simulink model "LQR_sim_with_equations_of_motion"  (R2022b)
settings: Solver=VariableStepAuto  StartTime=0.0  StopTime=10  RelTol=1e-3
undefined symbols (not defined in the file or in its folder): DiscIntNeverNeededParam, K
settings Model: Creator=Edvin  LastModifiedBy=Edvin

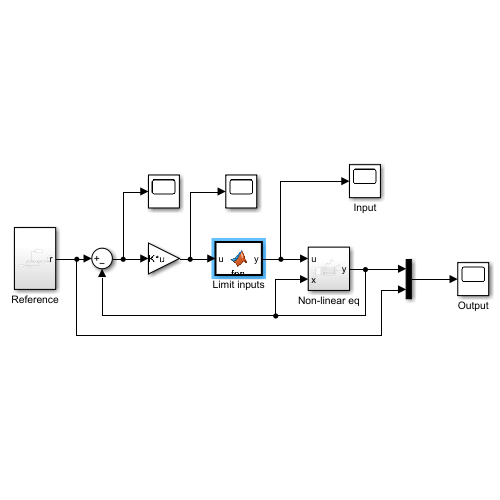
[thumbnail: Simulink's stored preview of the top-level diagram]
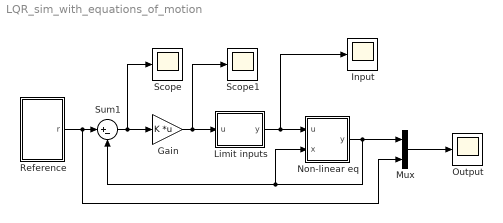
== system LQR_sim_with_equations_of_motion ==
  Gain : Gain  Gain=K  Multiplication=Matrix(K*u)
  Input : Scope
  Limit inputs : MATLAB Function  TreatAsAtomicUnit=on
  Mux : Mux  Inputs=2
  Non-linear eq : Subsystem
  Output : Scope
  Reference : Subsystem
  Scope : Scope
  Scope1 : Scope
  Sum1 : Sum  Inputs=|+-
  wires:
  Sum1/1 -> Scope/1, Gain/1
  Mux/1 -> Output/1
  Non-linear eq/1(y) -> Sum1/2, Non-linear eq/2(x), Mux/1
  Gain/1 -> Scope1/1, Limit inputs/1(u)
  Reference/1(r) -> Mux/2, Sum1/1
  Limit inputs/1(y) -> Input/1, Non-linear eq/1(u)

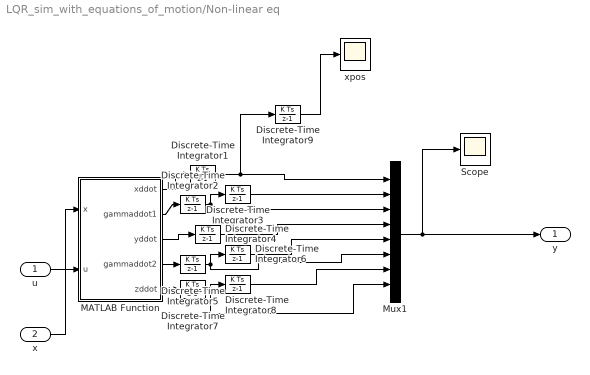
== system LQR_sim_with_equations_of_motion/Non-linear eq ==
  u : Inport
  x : Inport  Port=2
  Discrete-Time Integrator{1..9} (9 alike) : DiscreteIntegrator  SampleTime=-1  ICPrevOutput=DiscIntNeverNeededParam  ICPrevScaledInput=DiscIntNeverNeededParam
  MATLAB Function : MATLAB Function  TreatAsAtomicUnit=on
  Mux1 : Mux  Inputs=8
  Scope : Scope
  xpos : Scope
  y : Outport
  wires:
  MATLAB Function/1(xddot) -> Discrete-Time Integrator1/1
  u/1 -> MATLAB Function/2(u)
  Discrete-Time Integrator2/1 -> Mux1/3, Discrete-Time Integrator3/1
  MATLAB Function/2(gammaddot1) -> Discrete-Time Integrator2/1
  Discrete-Time Integrator6/1 -> Mux1/5
  MATLAB Function/3(yddot) -> Discrete-Time Integrator4/1
  Discrete-Time Integrator1/1 -> Discrete-Time Integrator9/1, Mux1/1
  MATLAB Function/5(zddot) -> Discrete-Time Integrator7/1
  Discrete-Time Integrator4/1 -> Mux1/4
  MATLAB Function/4(gammaddot2) -> Discrete-Time Integrator5/1
  Discrete-Time Integrator8/1 -> Mux1/7
  x/1 -> MATLAB Function/1(x)
  Discrete-Time Integrator5/1 -> Discrete-Time Integrator6/1, Mux1/6
  Discrete-Time Integrator3/1 -> Mux1/2
  Discrete-Time Integrator7/1 -> Discrete-Time Integrator8/1, Mux1/8
  Discrete-Time Integrator9/1 -> xpos/1
  Mux1/1 -> y/1, Scope/1

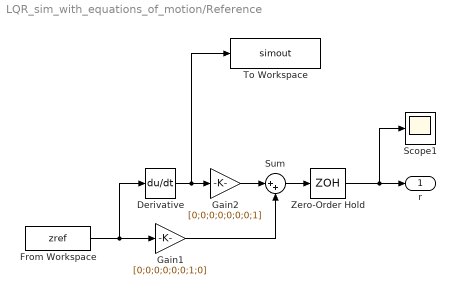
== system LQR_sim_with_equations_of_motion/Reference ==
  Derivative : Derivative
  From Workspace : FromWorkspace  VariableName=zref
  Gain1 : Gain  Gain=[0;0;0;0;0;0;1;0]
  Gain2 : Gain  Gain=[0;0;0;0;0;0;0;1]
  Scope1 : Scope
  Sum : Sum  Inputs=|++
  To Workspace : ToWorkspace  VariableName=simout  SampleTime=-1
      settings: Save2DSignal=2-D array (concatenate along first dimension)
  Zero-Order Hold : ZeroOrderHold  SampleTime=0.01
  r : Outport
  wires:
  Derivative/1 -> Gain2/1, To Workspace/1
  From Workspace/1 -> Derivative/1, Gain1/1
  Sum/1 -> Zero-Order Hold/1
  Gain1/1 -> Sum/2
  Gain2/1 -> Sum/1
  Zero-Order Hold/1 -> r/1, Scope1/1

== matlab function LQR_sim_with_equations_of_motion/Limit inputs ==
  data: u input; y output
function y = fcn(u)
g = 9.82; 
m = 2.5;
% Max thrust
Fmax = m*g;

% Calculate thrust
u(1) = m*g/2 + u(1);

% Limit thrust vector
if u(1) > Fmax
    u(1) = Fmax;
elseif u(1) <= 0 
    u(1) = 0;
end

% Limit gimble angles
if u(2) > 30
    u(2) = 30;
elseif u(2) < -30
    u(2) = -30;
end

if u(3) > 30
    u(3) = 30;
elseif u(3) < -30
    u(3) = -30;
end

y = u;

== matlab function LQR_sim_with_equations_of_motion/Non-linear eq/MATLAB Function ==
  data: x input; xddot output size=1; u input; gammaddot1 output size=1; yddot output size=1; gammaddot2 output size=1; zddot output size=1
function [xddot,gammaddot1,yddot,gammaddot2,zddot] = fcn(x,u)

Jx = 0.215;
Jy = 0.226;
h1 = 0.3;
h2 = 0.2;
h1 = 0.455933;
h2 = 0.330933;
g = 9.82;

m = 2.5;

Jx = 0.215;
Jy = 0.226;

%Rocket equations
xddot = u(1)/m * sind(x(2)+u(2));

gammaddot1 = u(1)*sind(u(2))*h1/Jy;

yddot = u(1)/m*sind(x(5)+u(3));

gammaddot2 = u(1)*sind(u(3))*h2/Jx;

zddot = u(1)*(cosd(x(2)+u(2))+cosd(x(5)+u(3)))/m-g;
